simulink library "dq_abc_lib_2011"  (Simulink 7.8)
settings: Solver=ode45  StartTime=0.0  StopTime=10.0  RelTol=1e-3
settings Model: Creator=CH24070  LastModifiedBy=CH24070

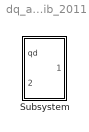
== system dq_abc_lib_2011 ==
  Subsystem : Subsystem

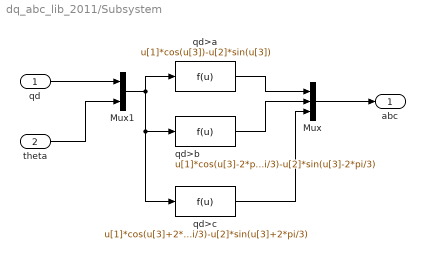
== system dq_abc_lib_2011/Subsystem ==
  qd : Inport  OutDataTypeStr=double  PortDimensions=2
  theta : Inport  Port=2  OutDataTypeStr=double  PortDimensions=1
  Mux : Mux  Inputs=3
  Mux1 : Mux  Inputs=2
  qd>a : Fcn  Expr=u[1]*cos(u[3])-u[2]*sin(u[3])
  qd>b : Fcn  Expr=u[1]*cos(u[3]-2*pi/3)-u[2]*sin(u[3]-2*pi/3)
  qd>c : Fcn  Expr=u[1]*cos(u[3]+2*pi/3)-u[2]*sin(u[3]+2*pi/3)
  abc : Outport  OutDataTypeStr=double  PortDimensions=3
  wires:
  Mux/1 -> abc/1
  qd>b/1 -> Mux/2
  qd/1 -> Mux1/1
  qd>c/1 -> Mux/3
  theta/1 -> Mux1/2
  Mux1/1 -> qd>c/1, qd>b/1, qd>a/1
  qd>a/1 -> Mux/1
